simulink model "pv_array"  (R2021a)
settings: Solver=VariableStepAuto  StartTime=0.0  StopTime=10.0  RelTol=1e-3
libraries: spsPVArrayLib x1, spsVoltageMeasurementLib x1, spspowerguiLib x1
settings Model: Creator=LENOVO  LastModifiedBy=LENOVO

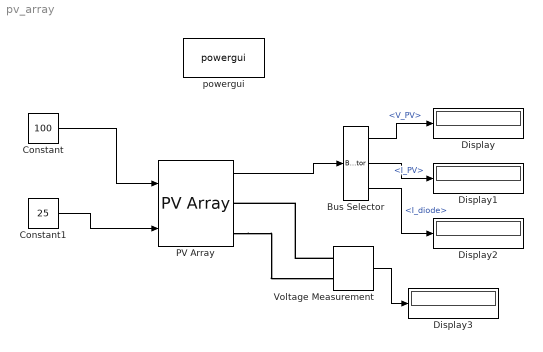
== system pv_array ==
  Bus Selector : BusSelector  OutputSignals=V_PV,I_PV,I_diode
  Constant : Constant  Value=100
  Constant1 : Constant  Value=25
  Display{,1..3} (4 alike) : Display
  PV Array : spsPVArrayLib/PV Array  Npar=40  Nser=10  PlotType=array @ 1000 W/m2 & specified temperatures  S_vec="[ 1000  500  100 ]"  Temp_C_vec="[ 45 25  ]"  ModuleName=Aavid Solar ASMS-165P  PlotWhenSelected=off  Pm=164.85  Ncell=72  Voc=43.5  Isc=5.25  Vm=35  Im=4.71  beta_Voc_pc=-0.393  alpha_Isc_pc=0.03  beta_Voc=-0.17095  alpha_Isc=0.001575  IL=5.2764  I0=4.9875e-10  nI=1.0218  Rsh=125.0069  Rs=0.62818  RobustModel=off  RobustCellTemperature=313.3991  BAL=on  Tc=1e-6  Tfilter=5e-5
      link override Diode Rsh/Transfer Fcn: Denominator=[1 1]
  Voltage Measurement : spsVoltageMeasurementLib/Voltage Measurement  PhasorSimulation=off  OutputType=Complex  PSBequivalent=0
  powergui : spspowerguiLib/powergui  Priority=1  SimulationMode=Continuous  SampleTime=50e-6  frequency=60  Iterations=50  frequencyindice=0  Pbase=100e6  ErrMax=1e-4  UnitsV=kV  UnitsW=MW  buscounter=0  FunctionMessages=off  echomessages=off  EnableUseOfTLC=off  CurrentSourceSwitches=off  DisableSnubberDevices=off  DisableRonSwitches=off  DisableVfSwitches=off  DisplayEquations=off  AutomaticDiscreteSolvers=off  SolverType=Tustin/Backward Euler (TBE)  Interpol=off  ExternalGateDelay=off  methode=off  Ts=100  x0status=blocks  SPID=on  SwTol=0  HookPort=off  NonlinearTolerance=1e-4  nMaxIteration=100  ContinueOnMaxIteration=off  RestoreLinks=warning  ResistiveCurrentMeasurement=off  Frange=[0:2:500]  Ylog=off  Xlog=on  ShowGrid=off  save=off  variable=ZData  structure=0  ZoomFFT=off  StartTime=0.0  cycles=1  DisplayStyle=1  fundamental=60  FreqAxis=off  MaxFrequency=1000  frequencyindicesteady=1  RmsSteady=1  display=off
  wires:
  Constant/1 -> PV Array/1
  Constant1/1 -> PV Array/2
  PV Array/1 -> Bus Selector/1
  Bus Selector/1 -> Display/1  "<V_PV>"
  Bus Selector/2 -> Display1/1  "<I_PV>"
  Bus Selector/3 -> Display2/1  "<I_diode>"
  Voltage Measurement/1 -> Display3/1
  connections:
  Voltage Measurement/LConn1 -- PV Array/RConn1
  PV Array/RConn2 -- Voltage Measurement/LConn2
